simulink model "SEPIC_PI"  (R2025a)
settings: Solver=FixedStepAuto  StartTime=0.0  StopTime=1  RelTol=1e-3
libraries: spsSeriesRLCBranchLib x5, spsVoltageMeasurementLib x3, spsGroundLib x2, spsDCVoltageSourceLib x1, spsCurrentMeasurementLib x1, spsDiodeLib x1, spsMosfetLib x1, simulink x1, spsVariableResistorLib x1, sps_lib x1
settings Model: Creator=gamezebra  LastModifiedBy=gamezebra

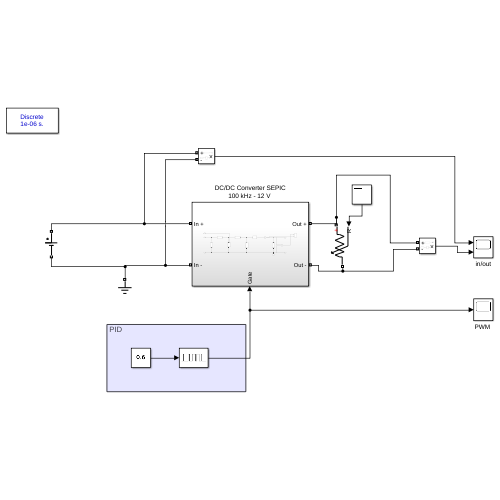
[thumbnail: Simulink's stored preview of the top-level diagram]
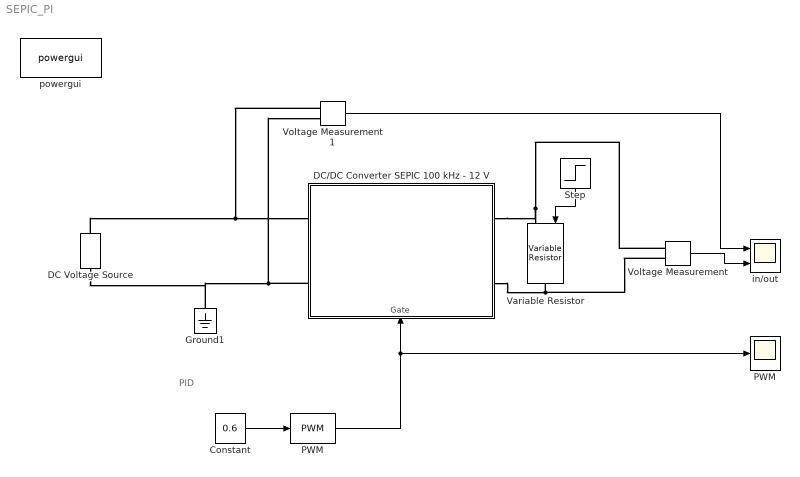
== system SEPIC_PI ==
  note: PID
  Constant : Constant  Value=0.6
  DC Voltage Source : spsDCVoltageSourceLib/DC Voltage Source  Amplitude=16.4  Measurements=None
  "DC/DC Converter SEPIC 100 kHz - 12 V " : Subsystem
      settings: PortSchema="{\"entries\":[{\"content\":{\"sides\":[{\"content\":{\"connectorIds\":[\"LConn1\",\"LConn2\"]},\"type\":\"ConnectorPlacement.EquallySpacedRectSide\",\"uuid\":\"91feb529-5820-4edf-8d0e-1c637fed9421\"},{\"content\":{\"connectorIds\":[\"RConn1\",\"RConn2\"],\"side\":\"RIGHT\"},\"type\":\"ConnectorPlacement.EquallySpacedRectSide\",\"uuid\":\"b4099113-c0ef-4c50-8083-88b14b98cc04\"},{\"content\":{\"side\":\"TOP\"},\"type\":\"ConnectorPlacement.EquallySpacedRectSide\",\"uuid\":\"250c6351-2de3-43d7-b6c9-3c3ed0452184\"},{\"content\":{\"connectorIds\":[\"In1\"],\"side\":\"BOTTOM\"},\"type\":\"ConnectorPlacement.EquallySpacedRectSide\",\"uuid\":\"484af620-bbf2-4328-991e-a08b15b59058\"}]},\"type\":\"ConnectorPlacement.EquallySpacedConnector\",\"uuid\":\"7041a545-1967-46d5-8643-e26f6c990daf\"}],\"packageUris\":[\"http://schema.mathworks.com/mf0/Connector/R2020b\"],\"version\":\"1.0\"}"
  Ground1 : spsGroundLib/Ground  LConnTagsString=a
  PWM : simulink/Discontinuities/PWM  DisableCoverage=on  Period=1/100000  InitialDelay=0  DisallowZeroDutyCycle=off  RunAtFixedTimeIntervals=on  SampleTime=0.000001
  "PWM " : Scope
      settings: Title=PWM  ActiveDisplayYMinimum=0.19673605992835486  ActiveDisplayYMaximum=1.3583645624515657  YLabel=Amplitudo
  Step : Step  Time=0.4  Before=20  After=10  SampleTime=0
  Variable Resistor : spsVariableResistorLib/Variable Resistor  Rabsmin=1e-3
      settings: LibrarySourceBlock=sps_lib/Passives/Variable Resistor
  Voltage Measurement : spsVoltageMeasurementLib/Voltage Measurement  PhasorSimulation=off  OutputType=Complex  PSBequivalent=0
  Voltage Measurement1 : spsVoltageMeasurementLib/Voltage Measurement  PhasorSimulation=off  OutputType=Complex  PSBequivalent=0
  in/out : Scope  NumInputPorts=2
      settings: Title=PWM  ActiveDisplayYMinimum=-5.7775896075635558  ActiveDisplayYMaximum=37.897884724058827  YLabel=Amplitudo  DataLoggingVariableName=ScopeData3
  powergui : sps_lib/powergui  Priority=1  SimulationMode=Discrete  SampleTime=0.000001  frequency=60  Iterations=50  frequencyindice=0  Pbase=100e6  ErrMax=1e-4  UnitsV=kV  UnitsW=MW  buscounter=0  FunctionMessages=off  echomessages=off  EnableUseOfTLC=off  CurrentSourceSwitches=off  DisableSnubberDevices=off  DisableRonSwitches=off  DisableVfSwitches=off  DisplayEquations=off  AutomaticDiscreteSolvers=off  SolverType=Tustin/Backward Euler (TBE)  Interpol=off  ExternalGateDelay=off  methode=off  Ts=100  x0status=blocks  SPID=on  SwTol=0  HookPort=off  NonlinearTolerance=1e-4  nMaxIteration=100  ContinueOnMaxIteration=off  RestoreLinks=warning  ResistiveCurrentMeasurement=off  Frange=[0:2:500]  Ylog=off  Xlog=on  ShowGrid=off  save=off  variable=ZData  structure=0  ZoomFFT=off  StartTime=0.0  cycles=1  DisplayStyle=1  fundamental=60  FreqAxis=off  MaxFrequency=1000  frequencyindicesteady=1  RmsSteady=1  display=off
  wires:
  Constant/1 -> PWM/1
  Voltage Measurement1/1 -> in/out/1
  Voltage Measurement/1 -> in/out/2
  PWM/1 -> "PWM "/1, "DC/DC Converter SEPIC 100 kHz - 12 V "/1(Gate)
  Step/1 -> Variable Resistor/1
  connections:
  Voltage Measurement1/LConn1 -- DC Voltage Source/RConn1 -- "DC/DC Converter SEPIC 100 kHz - 12 V "/LConn1
  "DC/DC Converter SEPIC 100 kHz - 12 V "/RConn1 -- Voltage Measurement/LConn1 -- Variable Resistor/LConn1
  "DC/DC Converter SEPIC 100 kHz - 12 V "/RConn2 -- Voltage Measurement/LConn2 -- Variable Resistor/RConn1
  "DC/DC Converter SEPIC 100 kHz - 12 V "/LConn2 -- Voltage Measurement1/LConn2 -- DC Voltage Source/LConn1 -- Ground1/LConn1

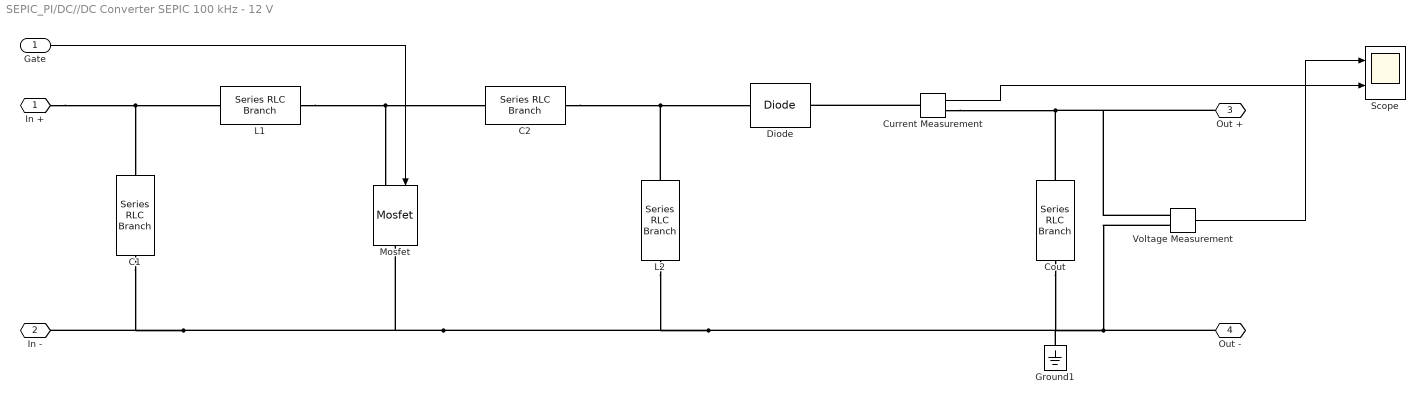
== system SEPIC_PI/DC//DC Converter SEPIC 100 kHz - 12 V  ==
  Gate : Inport
  C1 : spsSeriesRLCBranchLib/Series RLC Branch  LConnTagsString=__new0  RConnTagsString=__new0  BranchType=RC  Resistance=0.01  Inductance=1e-3  SetiL0=off  InitialCurrent=0  Capacitance=0.0001  Setx0=off  InitialVoltage=0  Measurements=None
  C2 : spsSeriesRLCBranchLib/Series RLC Branch  LConnTagsString=__new0  RConnTagsString=__new0  BranchType=C  Resistance=1  Inductance=1e-3  SetiL0=off  InitialCurrent=0  Capacitance=0.00001  Setx0=off  InitialVoltage=0  Measurements=None
  Cout : spsSeriesRLCBranchLib/Series RLC Branch  LConnTagsString=__new0  RConnTagsString=__new0  BranchType=RC  Resistance=0.01  Inductance=16.8e-3  SetiL0=off  InitialCurrent=0  Capacitance=0.0001  Setx0=off  InitialVoltage=0  Measurements=None
  "Current Measurement " : spsCurrentMeasurementLib/Current Measurement  PhasorSimulation=off  OutputType=Complex  PSBequivalent=0
  "Diode " : spsDiodeLib/Diode  Ron=0.001  Lon=0  Vf=0.5  IC=0  UseSnubber=0  Rs=500  Cs=250e-9  Measurements=off
  Ground1 : spsGroundLib/Ground  LConnTagsString=a
  L1 : spsSeriesRLCBranchLib/Series RLC Branch  LConnTagsString=__new0  RConnTagsString=__new0  BranchType=RL  Resistance=0.2  Inductance=0.0002  SetiL0=off  InitialCurrent=0  Capacitance=1e-6  Setx0=off  InitialVoltage=0  Measurements=None
  L2 : spsSeriesRLCBranchLib/Series RLC Branch  LConnTagsString=__new0  RConnTagsString=__new0  BranchType=RL  Resistance=0.2  Inductance=0.0002  SetiL0=off  InitialCurrent=0  Capacitance=1e-6  Setx0=off  InitialVoltage=0  Measurements=None
  Mosfet : spsMosfetLib/Mosfet  Ron=0.1  Lon=0  Rd=0.01  Vfd=0  IC=0  Rs=1e5  Cs=inf  Measurements=off
  Scope : Scope  NumInputPorts=2
      settings: Title=Tegangan Keluaran Konverter SEPIC  ActiveDisplayYMinimum=-151.86738214367281  ActiveDisplayYMaximum=1366.8064463408562  YLabel=Tegangan (Volts)
  "Voltage Measurement " : spsVoltageMeasurementLib/Voltage Measurement  PhasorSimulation=off  OutputType=Complex  PSBequivalent=0
  In + : PMIOPort  Side=Left
  In - : PMIOPort  Port=2  Side=Left
  Out + : PMIOPort  Port=3  Side=Right
  Out - : PMIOPort  Port=4  Side=Right
  wires:
  Gate/1 -> Mosfet/1
  "Current Measurement "/1 -> Scope/2
  "Voltage Measurement "/1 -> Scope/1
  connections:
  Out -/RConn1 -- Cout/RConn1 -- Ground1/LConn1 -- L2/RConn1 -- Mosfet/RConn1 -- C1/RConn1 -- In -/RConn1 -- "Voltage Measurement "/LConn2
  L1/RConn1 -- C2/LConn1 -- Mosfet/LConn1
  C2/RConn1 -- L2/LConn1 -- "Diode "/LConn1
  Cout/LConn1 -- "Voltage Measurement "/LConn1 -- Out +/RConn1 -- "Current Measurement "/RConn1
  In +/RConn1 -- L1/LConn1 -- C1/LConn1
  "Current Measurement "/LConn1 -- "Diode "/RConn1
